simulink subsystem "Leds"  (R2023b)
settings: Solver=VariableStepAuto  StartTime=0.0  StopTime=10.0  RelTol=1e-3
libraries: arduinolib x6, simulink x1
settings Model: Creator=Andrés  LastModifiedBy=Andrés

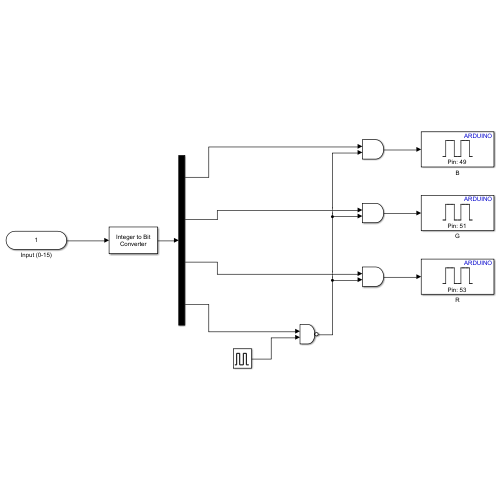
[thumbnail: Simulink's stored preview of the top-level diagram]
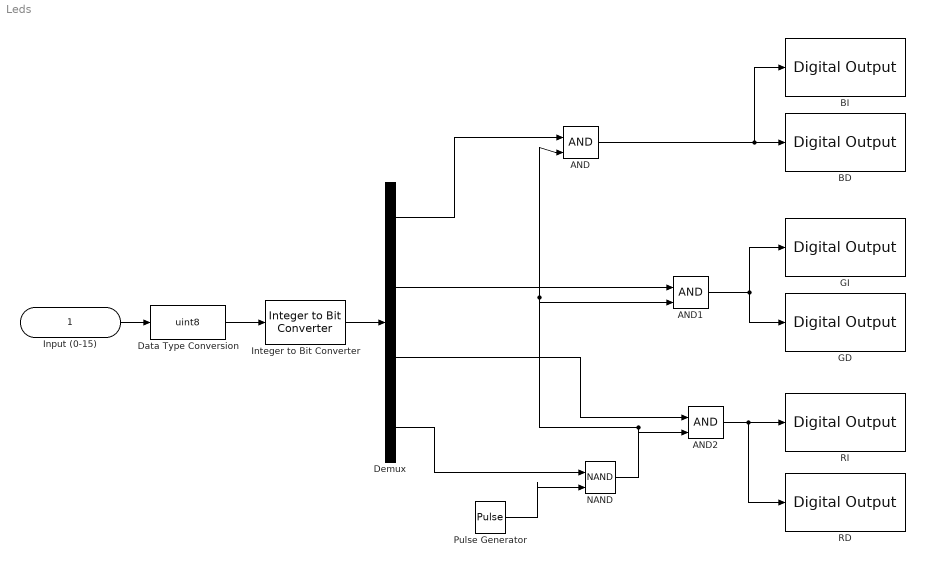
== system Leds ==
  Input (0-15) : Inport
  AND : Logic  IconShape=distinctive  AllPortsSameDT=off  OutDataTypeStr=boolean
  AND1 : Logic  IconShape=distinctive  AllPortsSameDT=off  OutDataTypeStr=boolean
  AND2 : Logic  IconShape=distinctive  AllPortsSameDT=off  OutDataTypeStr=boolean
  BD : arduinolib/Digital Output  pinNumber=10  Direction=output  blockPlatform=arduino
  BI : arduinolib/Digital Output  pinNumber=13  Direction=output  blockPlatform=arduino
  Data Type Conversion : DataTypeConversion  OutDataTypeStr=uint8  SaturateOnIntegerOverflow=off  RndMeth=Floor
  Demux : Demux
  GD : arduinolib/Digital Output  pinNumber=9  Direction=output  blockPlatform=arduino
  GI : arduinolib/Digital Output  pinNumber=12  Direction=output  blockPlatform=arduino
  Integer to Bit Converter : simulink/Logic and Bit Operations/Integer to Bit Converter  nbits=4  signedInputValues=Unsigned  bitOrder=LSB first  outDtype=Inherit via internal rule
  NAND : Logic  Operator=NAND  IconShape=distinctive  AllPortsSameDT=off  OutDataTypeStr=boolean
  Pulse Generator : DiscretePulseGenerator  PulseType=Time based  Period=0.5  PulseWidth=50
  RD : arduinolib/Digital Output  pinNumber=8  Direction=output  blockPlatform=arduino
  RI : arduinolib/Digital Output  pinNumber=11  Direction=output  blockPlatform=arduino
  wires:
  Pulse Generator/1 -> NAND/2
  Demux/4 -> NAND/1
  Integer to Bit Converter/1 -> Demux/1
  NAND/1 -> AND2/2, AND1/2, AND/2
  Input (0-15)/1 -> Data Type Conversion/1
  AND2/1 -> RI/1, RD/1
  Demux/3 -> AND2/1
  AND/1 -> BI/1, BD/1
  Demux/2 -> AND1/1
  AND1/1 -> GD/1, GI/1
  Demux/1 -> AND/1
  Data Type Conversion/1 -> Integer to Bit Converter/1
